simulink model "reaction_wheel_model"  (R2023b)
settings: Solver=VariableStepAuto  StartTime=0.0  StopTime=120  RelTol=1e-3
values from neighbouring files (symbols this model uses):
  beta = 28.5    [reaction_wheel.m]    (also in sat_reaction_wheels_aocs.m)
  desiredAttitude = [30; 50; 70]    [reaction_wheel.m]    (also in sat_reaction_wheels_aocs.m)
  desiredRate = [0.2; 0.2; 0.2]    [reaction_wheel.m]    (also in sat_reaction_wheels_aocs.m)
  disturbanceTorque = [10^-6; 10^-6; 10^-6]    [reaction_wheel.m]    (also in sat_reaction_wheels_aocs.m)
  initialAttitude = [0; 0; 0]    [reaction_wheel.m]    (also in sat_reaction_wheels_aocs.m)
  initialRate = [15; -15; 15]    [reaction_wheel.m]    (also in sat_reaction_wheels_aocs.m)
  kd = [1; 1; 1]    [reaction_wheel.m]    (also in sat_reaction_wheels_aocs.m)
  kp = [1; 1; 1]    [reaction_wheel.m]    (also in sat_reaction_wheels_aocs.m)
  maxTorqueReactionWheel = 0.015    [reaction_wheel.m]    (also in sat_reaction_wheels_aocs.m)
  moiReactionWheel = 0.00042    [reaction_wheel.m]    (also in sat_reaction_wheels_aocs.m)
  moiSatellite = [2.10 0.00 0.01 ... (first row only)    [reaction_wheel.m]    (also in sat_reaction_wheels_aocs.m)
libraries: simulink_extras x7, matrix_library x1
settings Model: Creator=yuvan  LastModifiedBy=yuvan

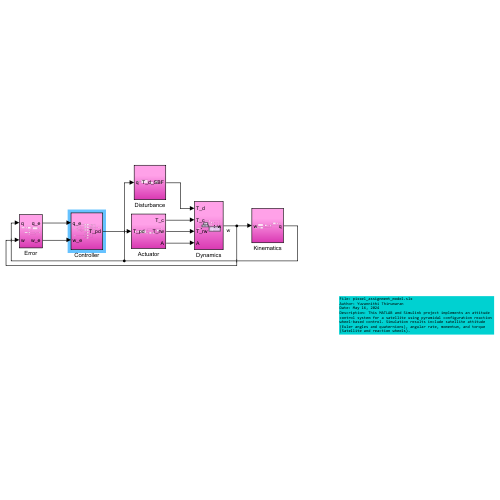
[thumbnail: Simulink's stored preview of the top-level diagram]
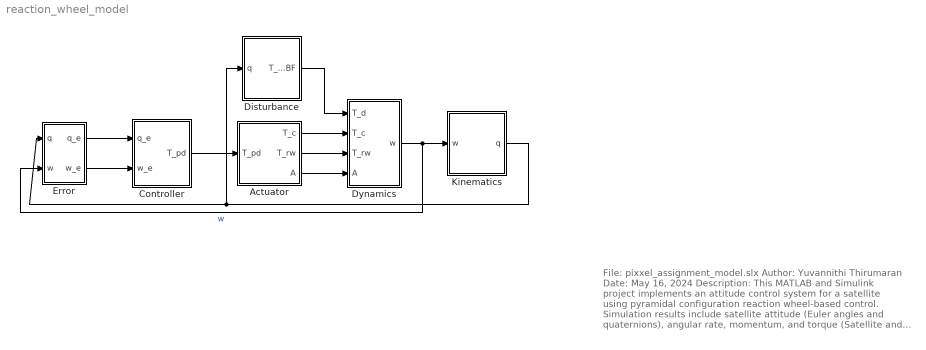
== system reaction_wheel_model ==
  note: File: pixxel_assignment_model.slx
      | Author: Yuvannithi Thirumaran
      | Date: May 16, 2024
      | Description: This MATLAB and Simulink project implements an attitude
      | control system for a satellite using pyramidal configuration reaction wheel-based control. Simulation results include satellite attitude (Euler angles and quaternions), angular rate, momentum, and torque (Satellite and reaction wheels).
  Actuator : Subsystem
  Controller : Subsystem
  Disturbance : Subsystem
  Dynamics : Subsystem
  Error : Subsystem
  Kinematics : Subsystem
  wires:
  Controller/1(T_pd) -> Actuator/1(T_pd)
  Kinematics/1(q) -> Error/1(q), Disturbance/1(q)
  Dynamics/1(w) -> Error/2(w), Kinematics/1(w)  "w"
  Actuator/1(T_c) -> Dynamics/2(T_c)
  Actuator/2(T_rw) -> Dynamics/3(T_rw)
  Actuator/3(A) -> Dynamics/4(A)
  Error/1(q_e) -> Controller/1(q_e)
  Disturbance/1(T_d_SBF) -> Dynamics/1(T_d)
  Error/2(w_e) -> Controller/2(w_e)

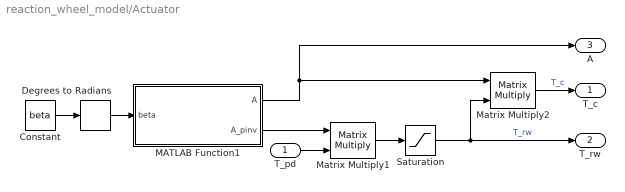
== system reaction_wheel_model/Actuator ==
  T_pd : Inport
  Constant : Constant  Value=beta
  Degrees to Radians : simulink_extras/Transformations/Degrees to Radians
  MATLAB Function1 : MATLAB Function  TreatAsAtomicUnit=on
  Matrix Multiply1 : Product  Multiplication=Matrix(*)
  Matrix Multiply2 : Product  Multiplication=Matrix(*)
  Saturation : Saturate  UpperLimit=maxTorqueReactionWheel  LowerLimit=-maxTorqueReactionWheel
  T_c : Outport
  T_rw : Outport  Port=2
  A : Outport  Port=3
  wires:
  Matrix Multiply2/1 -> T_c/1  "T_c"
  T_pd/1 -> Matrix Multiply1/2
  Constant/1 -> Degrees to Radians/1
  Saturation/1 -> Matrix Multiply2/2, T_rw/1  "T_rw"
  MATLAB Function1/1(A) -> A/1, Matrix Multiply2/1
  Matrix Multiply1/1 -> Saturation/1
  MATLAB Function1/2(A_pinv) -> Matrix Multiply1/1
  Degrees to Radians/1 -> MATLAB Function1/1(beta)

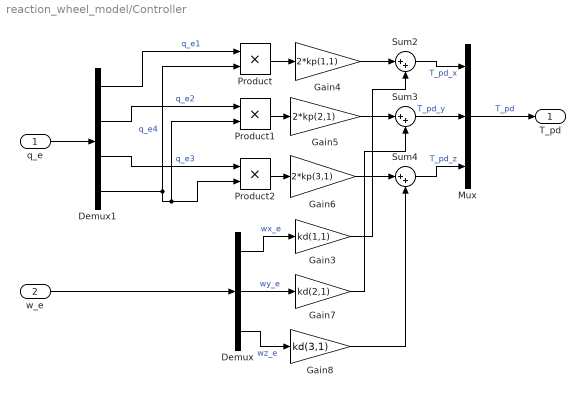
== system reaction_wheel_model/Controller ==
  q_e : Inport
  w_e : Inport  Port=2
  Demux : Demux  Outputs=3
  Demux1 : Demux
  Gain3 : Gain  Gain=kd(1,1)
  Gain4 : Gain  Gain=2*kp(1,1)
  Gain5 : Gain  Gain=2*kp(2,1)
  Gain6 : Gain  Gain=2*kp(3,1)
  Gain7 : Gain  Gain=kd(2,1)
  Gain8 : Gain  Gain=kd(3,1)
  Mux : Mux  Inputs=3
  Product : Product
  Product1 : Product
  Product2 : Product
  Sum2 : Sum  Inputs=|++
  Sum3 : Sum  Inputs=|++
  Sum4 : Sum  Inputs=|++
  T_pd : Outport
  wires:
  w_e/1 -> Demux/1
  Demux1/4 -> Product1/2, Product2/2, Product/2  "q_e4"
  Demux1/3 -> Product2/1  "q_e3"
  Demux1/2 -> Product1/1  "q_e2"
  Gain6/1 -> Sum4/1
  q_e/1 -> Demux1/1
  Demux1/1 -> Product/1  "q_e1"
  Product1/1 -> Gain5/1
  Product/1 -> Gain4/1
  Product2/1 -> Gain6/1
  Demux/1 -> Gain3/1  "wx_e"
  Demux/2 -> Gain7/1  "wy_e"
  Demux/3 -> Gain8/1  "wz_e"
  Gain4/1 -> Sum2/1
  Sum2/1 -> Mux/1  "T_pd_x"
  Gain5/1 -> Sum3/1
  Sum3/1 -> Mux/2  "T_pd_y"
  Sum4/1 -> Mux/3  "T_pd_z"
  Mux/1 -> T_pd/1  "T_pd"
  Gain3/1 -> Sum2/2
  Gain7/1 -> Sum3/2
  Gain8/1 -> Sum4/2

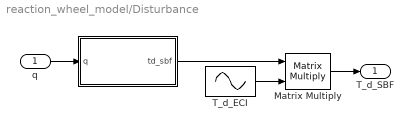
== system reaction_wheel_model/Disturbance ==
  q : Inport
  " " : MATLAB Function  TreatAsAtomicUnit=on
  Matrix Multiply : Product  Multiplication=Matrix(*)
  T_d_ECI : Sin  Amplitude=disturbanceTorque  SampleTime=0
  T_d_SBF : Outport
  wires:
  " "/1(td_sbf) -> Matrix Multiply/1
  Matrix Multiply/1 -> T_d_SBF/1
  q/1 -> " "/1(q)
  T_d_ECI/1 -> Matrix Multiply/2

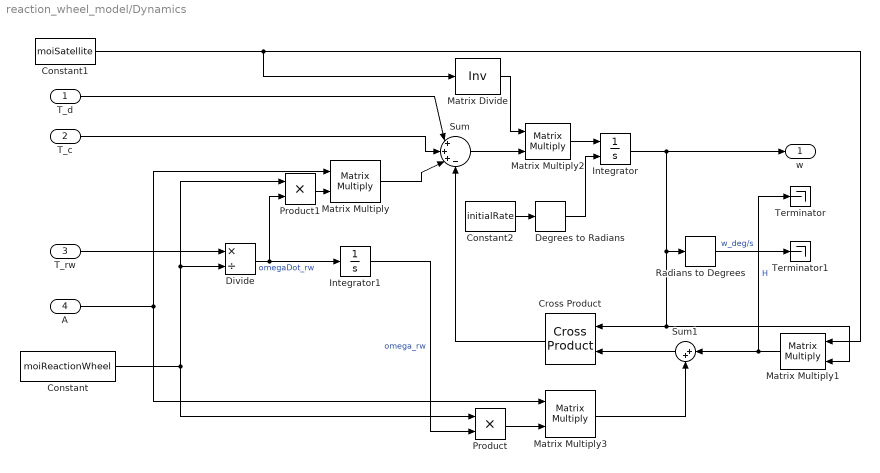
== system reaction_wheel_model/Dynamics ==
  T_d : Inport
  T_c : Inport  Port=2
  T_rw : Inport  Port=3
  A : Inport  Port=4
  Constant : Constant  Value=moiReactionWheel
  Constant1 : Constant  Value=moiSatellite
  Constant2 : Constant  Value=initialRate
  Cross Product : matrix_library/Cross Product
  Degrees to Radians : simulink_extras/Transformations/Degrees to Radians
  Divide : Product  Inputs=*/
  Integrator : Integrator  InitialConditionSource=external  InitialCondition=initialRate
  Integrator1 : Integrator  InitialCondition=zeros(4,1)
  Matrix Divide : Product  Inputs=/  Multiplication=Matrix(*)
  Matrix Multiply{,1..3} (4 alike) : Product  Multiplication=Matrix(*)
  Product : Product
  Product1 : Product
  Radians to Degrees : simulink_extras/Transformations/Radians to Degrees
  Sum : Sum  Inputs=|+++-
  Sum1 : Sum  Inputs=|++
  Terminator : Terminator
  Terminator1 : Terminator
  w : Outport
  wires:
  Integrator/1 -> w/1, Matrix Multiply1/2, Cross Product/1, Radians to Degrees/1
  Radians to Degrees/1 -> Terminator1/1  "w_deg/s"
  T_d/1 -> Sum/1
  T_c/1 -> Sum/2
  T_rw/1 -> Divide/1
  Constant/1 -> Product/1, Product1/1, Divide/2
  Divide/1 -> Integrator1/1, Product1/2  "omegaDot_rw"
  Matrix Multiply/1 -> Sum/3
  Cross Product/1 -> Sum/4
  Matrix Multiply1/1 -> Terminator/1, Sum1/1  "H"
  Constant1/1 -> Matrix Divide/1, Matrix Multiply1/1
  Matrix Multiply2/1 -> Integrator/1
  Sum/1 -> Matrix Multiply2/2
  Matrix Divide/1 -> Matrix Multiply2/1
  Matrix Multiply3/1 -> Sum1/2
  A/1 -> Matrix Multiply/1, Matrix Multiply3/1
  Integrator1/1 -> Product/2  "omega_rw"
  Product/1 -> Matrix Multiply3/2
  Product1/1 -> Matrix Multiply/2
  Sum1/1 -> Cross Product/2
  Degrees to Radians/1 -> Integrator/2
  Constant2/1 -> Degrees to Radians/1

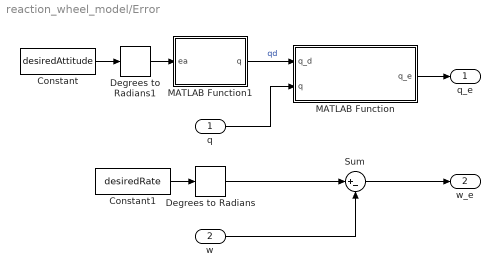
== system reaction_wheel_model/Error ==
  q : Inport
  w : Inport  Port=2
  Constant : Constant  Value=desiredAttitude
  Constant1 : Constant  Value=desiredRate
  Degrees to Radians : simulink_extras/Transformations/Degrees to Radians
  Degrees to Radians1 : simulink_extras/Transformations/Degrees to Radians
  MATLAB Function : MATLAB Function  TreatAsAtomicUnit=on
  MATLAB Function1 : MATLAB Function  TreatAsAtomicUnit=on
  Sum : Sum  Inputs=|+-
  q_e : Outport
  w_e : Outport  Port=2
  wires:
  q/1 -> MATLAB Function/2(q)
  MATLAB Function1/1(q) -> MATLAB Function/1(q_d)  "qd"
  MATLAB Function/1(q_e) -> q_e/1
  Sum/1 -> w_e/1
  w/1 -> Sum/2
  Constant1/1 -> Degrees to Radians/1
  Degrees to Radians/1 -> Sum/1
  Degrees to Radians1/1 -> MATLAB Function1/1(ea)
  Constant/1 -> Degrees to Radians1/1

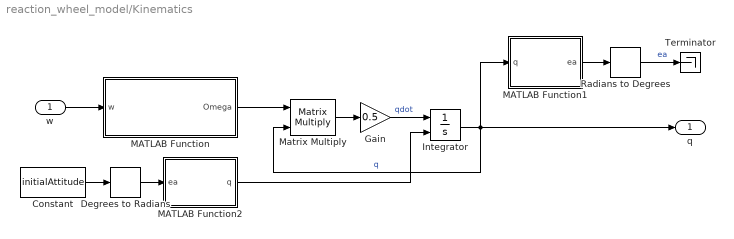
== system reaction_wheel_model/Kinematics ==
  w : Inport
  Constant : Constant  Value=initialAttitude
  Degrees to Radians : simulink_extras/Transformations/Degrees to Radians
  Gain : Gain  Gain=0.5
  Integrator : Integrator  InitialConditionSource=external  InitialCondition=[1; 0; 0; 0]
  MATLAB Function : MATLAB Function  TreatAsAtomicUnit=on
  MATLAB Function1 : MATLAB Function  TreatAsAtomicUnit=on
  MATLAB Function2 : MATLAB Function  TreatAsAtomicUnit=on
  Matrix Multiply : Product  Multiplication=Matrix(*)
  Radians to Degrees : simulink_extras/Transformations/Radians to Degrees
  Terminator : Terminator
  q : Outport
  wires:
  Matrix Multiply/1 -> Gain/1
  w/1 -> MATLAB Function/1(w)
  Integrator/1 -> Matrix Multiply/2, q/1, MATLAB Function1/1(q)  "q"
  MATLAB Function/1(Omega) -> Matrix Multiply/1
  Gain/1 -> Integrator/1  "qdot"
  MATLAB Function1/1(ea) -> Radians to Degrees/1
  Radians to Degrees/1 -> Terminator/1  "ea"
  Constant/1 -> Degrees to Radians/1
  MATLAB Function2/1(q) -> Integrator/2
  Degrees to Radians/1 -> MATLAB Function2/1(ea)

== matlab function reaction_wheel_model/Kinematics/MATLAB Function ==
  data: w input; Omega output
function Omega = fcn(w)

wx = w(1,1);
wy = w(2,1);
wz = w(3,1);

Omega = [0,  wz, -wy,  wx;
       -wz,   0,  wx, wy;
        wy, -wx,   0,  wz;
       -wx, -wy, -wz,  0];

== matlab function reaction_wheel_model/Actuator/MATLAB Function1 ==
  data: beta input; A output; A_pinv output
function [A, A_pinv] = configMatrix(beta)

A = [cos(beta) 0 -cos(beta) 0;
     0 cos(beta) 0 -cos(beta);
     sin(beta) sin(beta) sin(beta) sin(beta)];

A_pinv = pinv(A);

== matlab function reaction_wheel_model/Error/MATLAB Function1 ==
  data: ea input; q output
function q = fcn(ea)

phi = ea(1,1);
theta = ea(2,1);
psi = ea(3,1);

q1 =  sin(psi/2)*sin(theta/2)*sin(phi/2) + cos(psi/2)*cos(theta/2)*cos(phi/2);
q2 = -sin(psi/2)*sin(theta/2)*cos(phi/2) + cos(psi/2)*cos(theta/2)*sin(phi/2);
q3 =  sin(psi/2)*cos(theta/2)*sin(phi/2) + cos(psi/2)*sin(theta/2)*cos(phi/2);
q4 =  sin(psi/2)*cos(theta/2)*cos(phi/2) - cos(psi/2)*sin(theta/2)*sin(phi/2);

q = [q1; q2; q3; q4];

== matlab function reaction_wheel_model/Disturbance/  ==
  data: q input; td_sbf output
function td_sbf = eci2sbf(q)

q1 = q(1,1);
q2 = q(2,1);
q3 = q(3,1);
q4 = q(4,1);

td_sbf = [1 - 2*(q3^2 + q4^2),   2*(q2*q3 - q1*q4),   2*(q2*q4 + q1*q3);
            2*(q2*q3 + q1*q4), 1 - 2*(q2^2 + q4^2),   2*(q3*q4 - q1*q2);
            2*(q2*q4 - q1*q3),   2*(q3*q4 + q1*q2), 1 - 2*(q2^2 + q3^2)];

== matlab function reaction_wheel_model/Error/MATLAB Function ==
  data: q_d input; q_e output; q input
function q_e = quaternionError(q_d, q)

q_d1 = q_d(1,1);
q_d2 = q_d(2,1);
q_d3 = q_d(3,1);
q_d4 = q_d(4,1);

q_e = 0.5*[q_d4,  q_d3, -q_d2, q_d1;
          -q_d3,  q_d4,  q_d1, q_d2;
           q_d2, -q_d1,  q_d4, q_d3;
          -q_d1, -q_d2, -q_d3, q_d4]*[-q(1:3,1); q(4,1)];

== matlab function reaction_wheel_model/Kinematics/MATLAB Function1 ==
  data: ea output; q input
function ea = fcn(q)

q1 = q(1,1);
q2 = q(2,1);
q3 = q(3,1);
q4 = q(4,1);

phi = atan2(2*(q1*q2 + q3*q4), q1^2 - q2^2 - q3^2 + q4^2);
theta = -asin(2*(q2*q4 - q1*q3));
psi = atan2(2*(q1*q4 + q2*q3), q1^2 + q2^2 - q3^2 - q4^2);

ea = [phi; theta; psi];

== matlab function reaction_wheel_model/Kinematics/MATLAB Function2 ==
  data: ea input; q output
function q = fcn(ea)

phi = ea(1,1);
theta = ea(2,1);
psi = ea(3,1);

q1 =  sin(psi/2)*sin(theta/2)*sin(phi/2) + cos(psi/2)*cos(theta/2)*cos(phi/2);
q2 = -sin(psi/2)*sin(theta/2)*cos(phi/2) + cos(psi/2)*cos(theta/2)*sin(phi/2);
q3 =  sin(psi/2)*cos(theta/2)*sin(phi/2) + cos(psi/2)*sin(theta/2)*cos(phi/2);
q4 =  sin(psi/2)*cos(theta/2)*cos(phi/2) - cos(psi/2)*sin(theta/2)*sin(phi/2);

q = [q1; q2; q3; q4];
